simulink model "Second_Simulink"  (R2013a)
settings: Solver=ode45  StartTime=0.0  StopTime=10.0  RelTol=1e-3
settings Model: Creator=B407  LastModifiedBy=B407

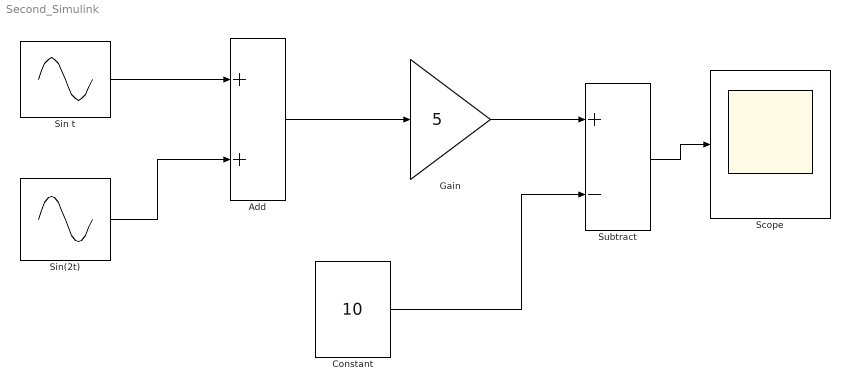
== system Second_Simulink ==
  Add : Sum
  Constant : Constant  Value=10
  Gain : Gain  Gain=5
  Scope : Scope
  Sin t : Sin  SampleTime=0
  Sin(2t) : Sin  Frequency=2  SampleTime=0
  Subtract : Sum  Inputs=+-
  wires:
  Gain/1 -> Subtract/1
  Sin t/1 -> Add/1
  Sin(2t)/1 -> Add/2
  Add/1 -> Gain/1
  Constant/1 -> Subtract/2
  Subtract/1 -> Scope/1
